simulink model "weather_task"  (Simulink 3.00)
libraries: mathlib x3, stringlib x2, analoglib x1

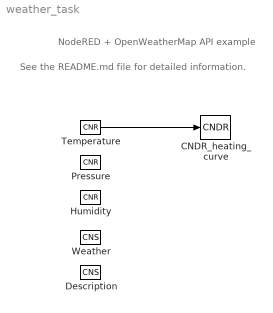
== system weather_task ==
  note: See the README.md file for detailed information.
  note: NodeRED + OpenWeatherMap API example
  CNDR_heating_curve : analoglib/CNDR  n=2  SATF=on  up=[-10 -5 0 5 10 15 20]  yp=[ 50 90 80 70 50 20 0 ]
  Description : stringlib/CNS  nmax=0
  Humidity : mathlib/CNR  ycn=1
  Pressure : mathlib/CNR  ycn=1
  Temperature : mathlib/CNR  ycn=1
  Weather : stringlib/CNS  nmax=0
  wires:
  Temperature/1 -> CNDR_heating_curve/1
